simulink model "main"  (R2025b)
settings: Solver=FixedStepDiscrete  StartTime=0.0  StopTime=Inf  RelTol=1e-3  EnableMultiTasking=on
PreLoadFcn:
  | RTWConfigurationCB('preloadfcn', bdroot);
model workspace (MAT data in the model file):
  fault_count = 0
  fz_values = [0 50 100 150 200 250 300 350 400 450 500 550 ... (43 elements, 1x43)]
  k_opt_lut = [0 0 0 0 0 0 0 0 0 0 0 0 ... (4386 elements, 51x2x43)]
  mu_opt_lut = [0 0 0 0 0 0 0 0 0 0 0 0 ... (4386 elements, 51x2x43)]
undefined symbols (not defined in the file or in its folder): bit, Call, Function, ocv_lut, slope_lut, soc_lut
libraries: c2837xDlib x34, c280xlib x20, canmsglib x18, c2802xlib x12, simulink x9, slpidlib x3
(part 2 of 5)

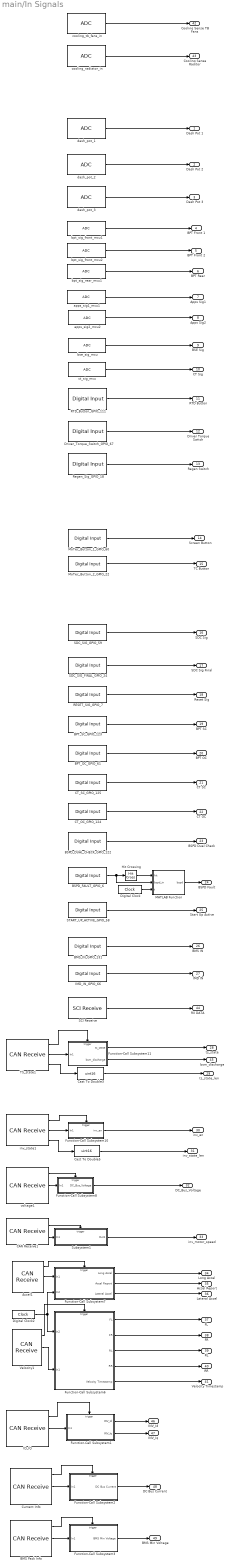
== system main/In Signals ==
  Accel1 : c280xlib/CAN Receive  chipFamily=C280x  useModule=CAN_B  mailboxNo=30  messageID=52  messageType=Standard (11-bit identifier)  enableAcceptanceFiltering=off  messageIDMask=0  sampleTime=.001  dataType=CAN_MESSAGE_TYPE  outputAction=Output last received values  initValue=0  outputMessageID=off  outputMessageLength=on  outputMessageTimeStamp=off  postInterrupt=off  interruptLine=0
  BMS Pack Info : c280xlib/CAN Receive  chipFamily=C280x  useModule=CAN_B  mailboxNo=21  messageID=237  messageType=Standard (11-bit identifier)  enableAcceptanceFiltering=off  messageIDMask=0  sampleTime=1.5  dataType=CAN_MESSAGE_TYPE  outputAction=Output last received values  initValue=2.8  outputMessageID=off  outputMessageLength=on  outputMessageTimeStamp=off  postInterrupt=off  interruptLine=0
  BMS_IN_GPIO_131 : c2837xDlib/Digital Input  GPIO_Number=GPIO128~GPIO135  GPIO_Bit0=off  GPIO_Bit1=off  GPIO_Bit2=off  GPIO_Bit3=on  GPIO_Bit4=off  GPIO_Bit5=off  GPIO_Bit6=off  GPIO_Bit7=off  sampleTime=0.01  dataType=auto  GPIO_Bit0_Qualification=Sync to SYSCLKOUT  GPIO_Bit1_Qualification=Sync to SYSCLKOUT  GPIO_Bit2_Qualification=Sync to SYSCLKOUT  GPIO_Bit3_Qualification=Sync to SYSCLKOUT  GPIO_Bit4_Qualification=Sync to SYSCLKOUT  GPIO_Bit5_Qualification=Sync to SYSCLKOUT  GPIO_Bit6_Qualification=Sync to SYSCLKOUT  GPIO_Bit7_Qualification=Sync to SYSCLKOUT  Qualification_Period=-1
  BPT_OC_GPIO_61 : c2837xDlib/Digital Input  GPIO_Number=GPIO56~GPIO63  GPIO_Bit0=off  GPIO_Bit1=off  GPIO_Bit2=off  GPIO_Bit3=off  GPIO_Bit4=off  GPIO_Bit5=on  GPIO_Bit6=off  GPIO_Bit7=off  sampleTime=0.01  dataType=auto  GPIO_Bit0_Qualification=Sync to SYSCLKOUT  GPIO_Bit1_Qualification=Sync to SYSCLKOUT  GPIO_Bit2_Qualification=Sync to SYSCLKOUT  GPIO_Bit3_Qualification=Sync to SYSCLKOUT  GPIO_Bit4_Qualification=Sync to SYSCLKOUT  GPIO_Bit5_Qualification=Sync to SYSCLKOUT  GPIO_Bit6_Qualification=Sync to SYSCLKOUT  GPIO_Bit7_Qualification=Sync to SYSCLKOUT  Qualification_Period=-1
  BPT_SC_GPIO_123 : c2837xDlib/Digital Input  GPIO_Number=GPIO120~GPIO127  GPIO_Bit0=off  GPIO_Bit1=off  GPIO_Bit2=off  GPIO_Bit3=on  GPIO_Bit4=off  GPIO_Bit5=off  GPIO_Bit6=off  GPIO_Bit7=off  sampleTime=0.01  dataType=auto  GPIO_Bit0_Qualification=Sync to SYSCLKOUT  GPIO_Bit1_Qualification=Sync to SYSCLKOUT  GPIO_Bit2_Qualification=Sync to SYSCLKOUT  GPIO_Bit3_Qualification=Sync to SYSCLKOUT  GPIO_Bit4_Qualification=Sync to SYSCLKOUT  GPIO_Bit5_Qualification=Sync to SYSCLKOUT  GPIO_Bit6_Qualification=Sync to SYSCLKOUT  GPIO_Bit7_Qualification=Sync to SYSCLKOUT  Qualification_Period=-1
  BSPD_DUAL_CHECK_GPIO_122 : c2837xDlib/Digital Input  GPIO_Number=GPIO120~GPIO127  GPIO_Bit0=off  GPIO_Bit1=off  GPIO_Bit2=on  GPIO_Bit3=off  GPIO_Bit4=off  GPIO_Bit5=off  GPIO_Bit6=off  GPIO_Bit7=off  sampleTime=0.01  dataType=auto  GPIO_Bit0_Qualification=Sync to SYSCLKOUT  GPIO_Bit1_Qualification=Sync to SYSCLKOUT  GPIO_Bit2_Qualification=Sync to SYSCLKOUT  GPIO_Bit3_Qualification=Sync to SYSCLKOUT  GPIO_Bit4_Qualification=Sync to SYSCLKOUT  GPIO_Bit5_Qualification=Sync to SYSCLKOUT  GPIO_Bit6_Qualification=Sync to SYSCLKOUT  GPIO_Bit7_Qualification=Sync to SYSCLKOUT  Qualification_Period=-1
  BSPD_FAULT_GPIO_6 : c2837xDlib/Digital Input  GPIO_Number=GPIO0~GPIO7  GPIO_Bit0=off  GPIO_Bit1=off  GPIO_Bit2=off  GPIO_Bit3=off  GPIO_Bit4=off  GPIO_Bit5=off  GPIO_Bit6=on  GPIO_Bit7=off  sampleTime=0.001  dataType=auto  GPIO_Bit0_Qualification=Sync to SYSCLKOUT  GPIO_Bit1_Qualification=Sync to SYSCLKOUT  GPIO_Bit2_Qualification=Sync to SYSCLKOUT  GPIO_Bit3_Qualification=Sync to SYSCLKOUT  GPIO_Bit4_Qualification=Sync to SYSCLKOUT  GPIO_Bit5_Qualification=Sync to SYSCLKOUT  GPIO_Bit6_Qualification=Sync to SYSCLKOUT  GPIO_Bit7_Qualification=Sync to SYSCLKOUT  Qualification_Period=-1
  CAN Receive1 : c280xlib/CAN Receive  chipFamily=C280x  useModule=CAN_B  mailboxNo=14  messageID=165  messageType=Standard (11-bit identifier)  enableAcceptanceFiltering=off  messageIDMask=0  sampleTime=0.003  dataType=CAN_MESSAGE_TYPE  outputAction=Output last received values  initValue=0  outputMessageID=off  outputMessageLength=off  outputMessageTimeStamp=off  postInterrupt=off  interruptLine=0
  CT_OC_GPIO_124 : c2837xDlib/Digital Input  GPIO_Number=GPIO120~GPIO127  GPIO_Bit0=off  GPIO_Bit1=off  GPIO_Bit2=off  GPIO_Bit3=off  GPIO_Bit4=on  GPIO_Bit5=off  GPIO_Bit6=off  GPIO_Bit7=off  sampleTime=0.01  dataType=auto  GPIO_Bit0_Qualification=Sync to SYSCLKOUT  GPIO_Bit1_Qualification=Sync to SYSCLKOUT  GPIO_Bit2_Qualification=Sync to SYSCLKOUT  GPIO_Bit3_Qualification=Sync to SYSCLKOUT  GPIO_Bit4_Qualification=Sync to SYSCLKOUT  GPIO_Bit5_Qualification=Sync to SYSCLKOUT  GPIO_Bit6_Qualification=Sync to SYSCLKOUT  GPIO_Bit7_Qualification=Sync to SYSCLKOUT  Qualification_Period=-1
  CT_SC_GPIO_125 : c2837xDlib/Digital Input  GPIO_Number=GPIO120~GPIO127  GPIO_Bit0=off  GPIO_Bit1=off  GPIO_Bit2=off  GPIO_Bit3=off  GPIO_Bit4=off  GPIO_Bit5=on  GPIO_Bit6=off  GPIO_Bit7=off  sampleTime=0.01  dataType=auto  GPIO_Bit0_Qualification=Sync to SYSCLKOUT  GPIO_Bit1_Qualification=Sync to SYSCLKOUT  GPIO_Bit2_Qualification=Sync to SYSCLKOUT  GPIO_Bit3_Qualification=Sync to SYSCLKOUT  GPIO_Bit4_Qualification=Sync to SYSCLKOUT  GPIO_Bit5_Qualification=Sync to SYSCLKOUT  GPIO_Bit6_Qualification=Sync to SYSCLKOUT  GPIO_Bit7_Qualification=Sync to SYSCLKOUT  Qualification_Period=-1
  Cast To Double3 : DataTypeConversion  OutDataTypeStr=uint16  SaturateOnIntegerOverflow=off  RndMeth=Floor
  Cast To Double5 : DataTypeConversion  OutDataTypeStr=uint16  SaturateOnIntegerOverflow=off  RndMeth=Floor
  Current Info : c280xlib/CAN Receive  chipFamily=C280x  useModule=CAN_B  mailboxNo=20  messageID=166  messageType=Standard (11-bit identifier)  enableAcceptanceFiltering=off  messageIDMask=0  sampleTime=0.003  dataType=CAN_MESSAGE_TYPE  outputAction=Reset all fields to zero  initValue=0  outputMessageID=off  outputMessageLength=on  outputMessageTimeStamp=off  postInterrupt=off  interruptLine=0
  Digital Clock : DigitalClock  SampleTime=0.001
  Digital Clock2 : DigitalClock  SampleTime=0.001
  Driver_Torque_Switch_GPIO_67 : c2837xDlib/Digital Input  GPIO_Number=GPIO64~GPIO71  GPIO_Bit0=off  GPIO_Bit1=off  GPIO_Bit2=off  GPIO_Bit3=on  GPIO_Bit4=off  GPIO_Bit5=off  GPIO_Bit6=off  GPIO_Bit7=off  sampleTime=0.1  dataType=single  GPIO_Bit0_Qualification=Sync to SYSCLKOUT  GPIO_Bit1_Qualification=Sync to SYSCLKOUT  GPIO_Bit2_Qualification=Sync to SYSCLKOUT  GPIO_Bit3_Qualification=Sync to SYSCLKOUT  GPIO_Bit4_Qualification=Sync to SYSCLKOUT  GPIO_Bit5_Qualification=Sync to SYSCLKOUT  GPIO_Bit6_Qualification=Sync to SYSCLKOUT  GPIO_Bit7_Qualification=Sync to SYSCLKOUT  Qualification_Period=-1
  Function-Call Subsystem1 : Subsystem  TreatAsAtomicUnit=on
  Function-Call Subsystem10 : Subsystem  TreatAsAtomicUnit=on
  Function-Call Subsystem11 : Subsystem  TreatAsAtomicUnit=on
  Function-Call Subsystem2 : Subsystem  TreatAsAtomicUnit=on
  Function-Call Subsystem3 : Subsystem  TreatAsAtomicUnit=on
  Function-Call Subsystem6 : Subsystem  TreatAsAtomicUnit=on
  Function-Call Subsystem7 : Subsystem  TreatAsAtomicUnit=on
  Function-Call Subsystem8 : Subsystem  TreatAsAtomicUnit=on
  Hit Crossing : HitCross  HitCrossingDirection=falling
  ID_IQ : c280xlib/CAN Receive  chipFamily=C280x  useModule=CAN_B  mailboxNo=19  messageID=168  messageType=Standard (11-bit identifier)  enableAcceptanceFiltering=off  messageIDMask=0  sampleTime=0.003  dataType=CAN_MESSAGE_TYPE  outputAction=Reset all fields to zero  initValue=0  outputMessageID=off  outputMessageLength=on  outputMessageTimeStamp=off  postInterrupt=off  interruptLine=0
  IMD_IN_GPIO_66 : c2837xDlib/Digital Input  GPIO_Number=GPIO64~GPIO71  GPIO_Bit0=off  GPIO_Bit1=off  GPIO_Bit2=on  GPIO_Bit3=off  GPIO_Bit4=off  GPIO_Bit5=off  GPIO_Bit6=off  GPIO_Bit7=off  sampleTime=0.01  dataType=auto  GPIO_Bit0_Qualification=Sync to SYSCLKOUT  GPIO_Bit1_Qualification=Sync to SYSCLKOUT  GPIO_Bit2_Qualification=Sync to SYSCLKOUT  GPIO_Bit3_Qualification=Sync to SYSCLKOUT  GPIO_Bit4_Qualification=Sync to SYSCLKOUT  GPIO_Bit5_Qualification=Sync to SYSCLKOUT  GPIO_Bit6_Qualification=Sync to SYSCLKOUT  GPIO_Bit7_Qualification=Sync to SYSCLKOUT  Qualification_Period=-1
  MATLAB Function : MATLAB Function  TreatAsAtomicUnit=on
  MoTec_Button_1_GPIO_60 : c2837xDlib/Digital Input  GPIO_Number=GPIO56~GPIO63  GPIO_Bit0=off  GPIO_Bit1=off  GPIO_Bit2=off  GPIO_Bit3=off  GPIO_Bit4=on  GPIO_Bit5=off  GPIO_Bit6=off  GPIO_Bit7=off  sampleTime=0.05  dataType=single  GPIO_Bit0_Qualification=Sync to SYSCLKOUT  GPIO_Bit1_Qualification=Sync to SYSCLKOUT  GPIO_Bit2_Qualification=Sync to SYSCLKOUT  GPIO_Bit3_Qualification=Sync to SYSCLKOUT  GPIO_Bit4_Qualification=Sync to SYSCLKOUT  GPIO_Bit5_Qualification=Sync to SYSCLKOUT  GPIO_Bit6_Qualification=Sync to SYSCLKOUT  GPIO_Bit7_Qualification=Sync to SYSCLKOUT  Qualification_Period=-1
  MoTec_Button_2_GPIO_22 : c2837xDlib/Digital Input  GPIO_Number=GPIO16~GPIO23  GPIO_Bit0=off  GPIO_Bit1=off  GPIO_Bit2=off  GPIO_Bit3=off  GPIO_Bit4=off  GPIO_Bit5=off  GPIO_Bit6=on  GPIO_Bit7=off  sampleTime=0.01  dataType=auto  GPIO_Bit0_Qualification=Sync to SYSCLKOUT  GPIO_Bit1_Qualification=Sync to SYSCLKOUT  GPIO_Bit2_Qualification=Sync to SYSCLKOUT  GPIO_Bit3_Qualification=Sync to SYSCLKOUT  GPIO_Bit4_Qualification=Sync to SYSCLKOUT  GPIO_Bit5_Qualification=Sync to SYSCLKOUT  GPIO_Bit6_Qualification=Sync to SYSCLKOUT  GPIO_Bit7_Qualification=Sync to SYSCLKOUT  Qualification_Period=-1
  RESET_SIG_GPIO_7 : c2837xDlib/Digital Input  GPIO_Number=GPIO0~GPIO7  GPIO_Bit0=off  GPIO_Bit1=off  GPIO_Bit2=off  GPIO_Bit3=off  GPIO_Bit4=off  GPIO_Bit5=off  GPIO_Bit6=off  GPIO_Bit7=on  sampleTime=0.01  dataType=auto  GPIO_Bit0_Qualification=Sync to SYSCLKOUT  GPIO_Bit1_Qualification=Sync to SYSCLKOUT  GPIO_Bit2_Qualification=Sync to SYSCLKOUT  GPIO_Bit3_Qualification=Sync to SYSCLKOUT  GPIO_Bit4_Qualification=Sync to SYSCLKOUT  GPIO_Bit5_Qualification=Sync to SYSCLKOUT  GPIO_Bit6_Qualification=Sync to SYSCLKOUT  GPIO_Bit7_Qualification=Sync to SYSCLKOUT  Qualification_Period=-1
  RTD_Button_GPIO_111 : c2837xDlib/Digital Input  GPIO_Number=GPIO104~GPIO111  GPIO_Bit0=off  GPIO_Bit1=off  GPIO_Bit2=off  GPIO_Bit3=off  GPIO_Bit4=off  GPIO_Bit5=off  GPIO_Bit6=off  GPIO_Bit7=on  sampleTime=0.1  dataType=single  GPIO_Bit0_Qualification=Sync to SYSCLKOUT  GPIO_Bit1_Qualification=Sync to SYSCLKOUT  GPIO_Bit2_Qualification=Sync to SYSCLKOUT  GPIO_Bit3_Qualification=Sync to SYSCLKOUT  GPIO_Bit4_Qualification=Sync to SYSCLKOUT  GPIO_Bit5_Qualification=Sync to SYSCLKOUT  GPIO_Bit6_Qualification=Sync to SYSCLKOUT  GPIO_Bit7_Qualification=Sync to SYSCLKOUT  Qualification_Period=-1
  Regen_Sig_GPIO_18 : c2837xDlib/Digital Input  GPIO_Number=GPIO16~GPIO23  GPIO_Bit0=off  GPIO_Bit1=off  GPIO_Bit2=on  GPIO_Bit3=off  GPIO_Bit4=off  GPIO_Bit5=off  GPIO_Bit6=off  GPIO_Bit7=off  sampleTime=0.01  dataType=single  GPIO_Bit0_Qualification=Sync to SYSCLKOUT  GPIO_Bit1_Qualification=Sync to SYSCLKOUT  GPIO_Bit2_Qualification=Sync to SYSCLKOUT  GPIO_Bit3_Qualification=Sync to SYSCLKOUT  GPIO_Bit4_Qualification=Sync to SYSCLKOUT  GPIO_Bit5_Qualification=Sync to SYSCLKOUT  GPIO_Bit6_Qualification=Sync to SYSCLKOUT  GPIO_Bit7_Qualification=Sync to SYSCLKOUT  Qualification_Period=-1
  SCI Receive : c280xlib/SCI Receive  Priority=2  sciModule=C  dataHead='S'  headerCheckMaxCount=16  dataTail='E'  dataType=int8  dataLenOptions=Length via dialog  dataDim=1  maxDataLength=1  initValue=0  errOption=Output the last received value  errValue=0  sampleTime=0.01  blockingMode=off  timeOut=inf  outputStatus=off
      settings: LibrarySourceBlock=c2802xlib/SCI Receive
  SDC_SIG_FINAL_GPIO_24 : c2837xDlib/Digital Input  GPIO_Number=GPIO24~GPIO31  GPIO_Bit0=on  GPIO_Bit1=off  GPIO_Bit2=off  GPIO_Bit3=off  GPIO_Bit4=off  GPIO_Bit5=off  GPIO_Bit6=off  GPIO_Bit7=off  sampleTime=0.001  dataType=auto  GPIO_Bit0_Qualification=Sync to SYSCLKOUT  GPIO_Bit1_Qualification=Sync to SYSCLKOUT  GPIO_Bit2_Qualification=Sync to SYSCLKOUT  GPIO_Bit3_Qualification=Sync to SYSCLKOUT  GPIO_Bit4_Qualification=Sync to SYSCLKOUT  GPIO_Bit5_Qualification=Sync to SYSCLKOUT  GPIO_Bit6_Qualification=Sync to SYSCLKOUT  GPIO_Bit7_Qualification=Sync to SYSCLKOUT  Qualification_Period=-1
  SDC_SIG_GPIO_59 : c2837xDlib/Digital Input  GPIO_Number=GPIO56~GPIO63  GPIO_Bit0=off  GPIO_Bit1=off  GPIO_Bit2=off  GPIO_Bit3=on  GPIO_Bit4=off  GPIO_Bit5=off  GPIO_Bit6=off  GPIO_Bit7=off  sampleTime=0.001  dataType=auto  GPIO_Bit0_Qualification=Sync to SYSCLKOUT  GPIO_Bit1_Qualification=Sync to SYSCLKOUT  GPIO_Bit2_Qualification=Sync to SYSCLKOUT  GPIO_Bit3_Qualification=Sync to SYSCLKOUT  GPIO_Bit4_Qualification=Sync to SYSCLKOUT  GPIO_Bit5_Qualification=Sync to SYSCLKOUT  GPIO_Bit6_Qualification=Sync to SYSCLKOUT  GPIO_Bit7_Qualification=Sync to SYSCLKOUT  Qualification_Period=-1
  START_UP_ACTIVE_GPIO_58 : c2837xDlib/Digital Input  GPIO_Number=GPIO56~GPIO63  GPIO_Bit0=off  GPIO_Bit1=off  GPIO_Bit2=on  GPIO_Bit3=off  GPIO_Bit4=off  GPIO_Bit5=off  GPIO_Bit6=off  GPIO_Bit7=off  sampleTime=0.01  dataType=auto  GPIO_Bit0_Qualification=Sync to SYSCLKOUT  GPIO_Bit1_Qualification=Sync to SYSCLKOUT  GPIO_Bit2_Qualification=Sync to SYSCLKOUT  GPIO_Bit3_Qualification=Sync to SYSCLKOUT  GPIO_Bit4_Qualification=Sync to SYSCLKOUT  GPIO_Bit5_Qualification=Sync to SYSCLKOUT  GPIO_Bit6_Qualification=Sync to SYSCLKOUT  GPIO_Bit7_Qualification=Sync to SYSCLKOUT  Qualification_Period=-1
  Subsystem1 : Subsystem
  TS_state1 : c280xlib/CAN Receive  chipFamily=C280x  useModule=CAN_B  mailboxNo=2  messageID=2  messageType=Standard (11-bit identifier)  enableAcceptanceFiltering=off  messageIDMask=0  sampleTime=.01  dataType=CAN_MESSAGE_TYPE  outputAction=Reset all fields to zero  initValue=0  outputMessageID=off  outputMessageLength=on  outputMessageTimeStamp=off  postInterrupt=off  interruptLine=0
  Velocity1 : c280xlib/CAN Receive  chipFamily=C280x  useModule=CAN_B  mailboxNo=9  messageID=51  messageType=Standard (11-bit identifier)  enableAcceptanceFiltering=off  messageIDMask=0  sampleTime=.001  dataType=CAN_MESSAGE_TYPE  outputAction=Output last received values  initValue=0  outputMessageID=off  outputMessageLength=on  outputMessageTimeStamp=off  postInterrupt=off  interruptLine=0
  apps_sig1_mcu1 : c2802xlib/ADC  blkParamProc=C2000_Type4  ADCModule=B  samplingMode=Single sample mode  ADCResolution=12-bit (Single-ended input)  ADC29xResolution=12-bit  ADCMode=Single-ended input  useSOC1=SOC6  useSOC2=SOC0_SOC1  SOCAcquisitionWindow=60  SOCTriggerSource=Software  SOCInterruptTrigger=No ADCINT  Ts=0.001  dType=uint16  postInterrupt=off  interruptSel=ADCINT1  ADCINTContinuous=on  endma=off  chdma=1  conv1=ADCINA0  conv2=ADCINA0 and ADCINB0  conv1_Type4=ADCIN3  conv2_Type4=ADCIN0 and ADCIN1
  apps_sig2_mcu2 : c2802xlib/ADC  blkParamProc=C2000_Type4  ADCModule=C  samplingMode=Single sample mode  ADCResolution=12-bit (Single-ended input)  ADC29xResolution=12-bit  ADCMode=Single-ended input  useSOC1=SOC7  useSOC2=SOC0_SOC1  SOCAcquisitionWindow=60  SOCTriggerSource=Software  SOCInterruptTrigger=No ADCINT  Ts=0.001  dType=uint16  postInterrupt=off  interruptSel=ADCINT1  ADCINTContinuous=on  endma=off  chdma=1  conv1=ADCINA0  conv2=ADCINA0 and ADCINB0  conv1_Type4=ADCIN3  conv2_Type4=ADCIN0 and ADCIN1
  bpt_sig_front_mcu1 : c2802xlib/ADC  blkParamProc=C2000_Type4  ADCModule=B  samplingMode=Single sample mode  ADCResolution=12-bit (Single-ended input)  ADC29xResolution=12-bit  ADCMode=Single-ended input  useSOC1=SOC3  useSOC2=SOC0_SOC1  SOCAcquisitionWindow=60  SOCTriggerSource=Software  SOCInterruptTrigger=No ADCINT  Ts=0.001  dType=uint16  postInterrupt=off  interruptSel=ADCINT1  ADCINTContinuous=on  endma=off  chdma=1  conv1=ADCINA0  conv2=ADCINA0 and ADCINB0  conv1_Type4=ADCIN4  conv2_Type4=ADCIN0 and ADCIN1
  bpt_sig_front_mcu2 : c2802xlib/ADC  blkParamProc=C2000_Type4  ADCModule=B  samplingMode=Single sample mode  ADCResolution=12-bit (Single-ended input)  ADC29xResolution=12-bit  ADCMode=Single-ended input  useSOC1=SOC4  useSOC2=SOC0_SOC1  SOCAcquisitionWindow=60  SOCTriggerSource=Software  SOCInterruptTrigger=No ADCINT  Ts=0.001  dType=uint16  postInterrupt=off  interruptSel=ADCINT1  ADCINTContinuous=on  endma=off  chdma=1  conv1=ADCINA0  conv2=ADCINA0 and ADCINB0  conv1_Type4=ADCIN2  conv2_Type4=ADCIN0 and ADCIN1
  bpt_sig_rear_mcu1 : c2802xlib/ADC  blkParamProc=C2000_Type4  ADCModule=C  samplingMode=Single sample mode  ADCResolution=12-bit (Single-ended input)  ADC29xResolution=12-bit  ADCMode=Single-ended input  useSOC1=SOC5  useSOC2=SOC0_SOC1  SOCAcquisitionWindow=60  SOCTriggerSource=Software  SOCInterruptTrigger=No ADCINT  Ts=0.001  dType=uint16  postInterrupt=off  interruptSel=ADCINT1  ADCINTContinuous=on  endma=off  chdma=1  conv1=ADCINA0  conv2=ADCINA0 and ADCINB0  conv1_Type4=ADCIN2  conv2_Type4=ADCIN0 and ADCIN1
  bse_sig_mcu : c2802xlib/ADC  blkParamProc=C2000_Type4  ADCModule=A  samplingMode=Single sample mode  ADCResolution=12-bit (Single-ended input)  ADC29xResolution=12-bit  ADCMode=Single-ended input  useSOC1=SOC8  useSOC2=SOC0_SOC1  SOCAcquisitionWindow=60  SOCTriggerSource=Software  SOCInterruptTrigger=No ADCINT  Ts=0.01  dType=uint16  postInterrupt=off  interruptSel=ADCINT1  ADCINTContinuous=on  endma=off  chdma=1  conv1=ADCINA0  conv2=ADCINA0 and ADCINB0  conv1_Type4=ADCIN3  conv2_Type4=ADCIN0 and ADCIN1
  cooling_radiator_in : c2802xlib/ADC  blkParamProc=C2000_Type4  ADCModule=A  samplingMode=Single sample mode  ADCResolution=12-bit (Single-ended input)  ADC29xResolution=12-bit  ADCMode=Single-ended input  useSOC1=SOC11  useSOC2=SOC0_SOC1  SOCAcquisitionWindow=60  SOCTriggerSource=Software  SOCInterruptTrigger=ADCINT1  Ts=1  dType=uint16  postInterrupt=off  interruptSel=ADCINT1  ADCINTContinuous=on  endma=off  chdma=1  conv1=ADCINA0  conv2=ADCINA0 and ADCINB0  conv1_Type4=ADCIN5  conv2_Type4=ADCIN0 and ADCIN1
  cooling_tb_fans_in : c2802xlib/ADC  blkParamProc=C2000_Type4  ADCModule=B  samplingMode=Single sample mode  ADCResolution=12-bit (Single-ended input)  ADC29xResolution=12-bit  ADCMode=Single-ended input  useSOC1=SOC10  useSOC2=SOC0_SOC1  SOCAcquisitionWindow=60  SOCTriggerSource=Software  SOCInterruptTrigger=No ADCINT  Ts=1  dType=uint16  postInterrupt=off  interruptSel=ADCINT1  ADCINTContinuous=on  endma=off  chdma=1  conv1=ADCINA0  conv2=ADCINA0 and ADCINB0  conv1_Type4=ADCIN5  conv2_Type4=ADCIN0 and ADCIN1
  ct_sig_mcu : c2802xlib/ADC  blkParamProc=C2000_Type4  ADCModule=A  samplingMode=Single sample mode  ADCResolution=12-bit (Single-ended input)  ADC29xResolution=12-bit  ADCMode=Single-ended input  useSOC1=SOC9  useSOC2=SOC0_SOC1  SOCAcquisitionWindow=60  SOCTriggerSource=Software  SOCInterruptTrigger=No ADCINT  Ts=0.01  dType=uint16  postInterrupt=off  interruptSel=ADCINT1  ADCINTContinuous=on  endma=off  chdma=1  conv1=ADCINA0  conv2=ADCINA0 and ADCINB0  conv1_Type4=ADCIN2  conv2_Type4=ADCIN0 and ADCIN1
  dash_pot_1 : c2802xlib/ADC  blkParamProc=C2000_Type4  ADCModule=A  samplingMode=Single sample mode  ADCResolution=12-bit (Single-ended input)  ADC29xResolution=12-bit  ADCMode=Single-ended input  useSOC1=SOC0  useSOC2=SOC0_SOC1  SOCAcquisitionWindow=60  SOCTriggerSource=Software  SOCInterruptTrigger=No ADCINT  Ts=0.05  dType=uint16  postInterrupt=off  interruptSel=ADCINT1  ADCINTContinuous=on  endma=off  chdma=1  conv1=ADCINA0  conv2=ADCINA0 and ADCINB0  conv1_Type4=ADCIN14  conv2_Type4=ADCIN0 and ADCIN1
  dash_pot_2 : c2802xlib/ADC  blkParamProc=C2000_Type4  ADCModule=A  samplingMode=Single sample mode  ADCResolution=12-bit (Single-ended input)  ADC29xResolution=12-bit  ADCMode=Single-ended input  useSOC1=SOC1  useSOC2=SOC0_SOC1  SOCAcquisitionWindow=60  SOCTriggerSource=Software  SOCInterruptTrigger=No ADCINT  Ts=0.05  dType=uint16  postInterrupt=off  interruptSel=ADCINT1  ADCINTContinuous=on  endma=off  chdma=1  conv1=ADCINA0  conv2=ADCINA0 and ADCINB0  conv1_Type4=ADCIN4  conv2_Type4=ADCIN0 and ADCIN1
  dash_pot_3 : c2802xlib/ADC  blkParamProc=C2000_Type4  ADCModule=A  samplingMode=Single sample mode  ADCResolution=12-bit (Single-ended input)  ADC29xResolution=12-bit  ADCMode=Single-ended input  useSOC1=SOC2  useSOC2=SOC0_SOC1  SOCAcquisitionWindow=60  SOCTriggerSource=Software  SOCInterruptTrigger=No ADCINT  Ts=0.05  dType=uint16  postInterrupt=off  interruptSel=ADCINT1  ADCINTContinuous=on  endma=off  chdma=1  conv1=ADCINA0  conv2=ADCINA0 and ADCINB0  conv1_Type4=ADCIN1  conv2_Type4=ADCIN0 and ADCIN1
  inv_state1 : c280xlib/CAN Receive  chipFamily=C280x  useModule=CAN_B  mailboxNo=5  messageID=170  messageType=Standard (11-bit identifier)  enableAcceptanceFiltering=off  messageIDMask=0  sampleTime=.01  dataType=CAN_MESSAGE_TYPE  outputAction=Reset all fields to zero  initValue=0  outputMessageID=off  outputMessageLength=on  outputMessageTimeStamp=off  postInterrupt=off  interruptLine=0
  voltage1 : c280xlib/CAN Receive  chipFamily=C280x  useModule=CAN_B  mailboxNo=15  messageID=167  messageType=Standard (11-bit identifier)  enableAcceptanceFiltering=off  messageIDMask=0  sampleTime=0.003  dataType=CAN_MESSAGE_TYPE  outputAction=Reset all fields to zero  initValue=0  outputMessageID=off  outputMessageLength=on  outputMessageTimeStamp=off  postInterrupt=off  interruptLine=0
  Dash Pot 1 : Outport
  Dash Pot 2 : Outport  Port=2
  Dash Pot 3 : Outport  Port=3
  BPT Front 1 : Outport  Port=4
  BPT Front 2 : Outport  Port=5
  BPT Rear : Outport  Port=6
  Apps Sig1 : Outport  Port=7
  Apps Sig2 : Outport  Port=8
  BSE Sig : Outport  Port=9
  CT Sig : Outport  Port=10
  RTD Button : Outport  Port=11
  Driver Torque Switch : Outport  Port=12
  Regen Switch : Outport  Port=13
  Screen Button : Outport  Port=14
  TC Button : Outport  Port=15
  SDC Sig : Outport  Port=16
  SDC Sig Final : Outport  Port=17
  Reset Sig : Outport  Port=18
  BPT SC : Outport  Port=19
  BPT OC : Outport  Port=20
  CT SC : Outport  Port=21
  CT OC : Outport  Port=22
  BSPD Dual Check : Outport  Port=23
  BSPD Fault : Outport  Port=24
  Start Up Active : Outport  Port=25
  BMS IN : Outport  Port=26
  IMD IN : Outport  Port=27
  ts_state : Outport  Port=28
  ts_state_len : Outport  Port=29
  inv_en : Outport  Port=30
  inv_state_len : Outport  Port=31
  DC_Bus_Voltage : Outport  Port=32
  inv_motor_speed : Outport  Port=33
  Long Accel : Outport  Port=34
  Accel Report : Outport  Port=35
  Lateral Accel : Outport  Port=36
  FL : Outport  Port=37
  FR : Outport  Port=38
  RL : Outport  Port=39
  RR : Outport  Port=40
  Velocity Timestamp : Outport  Port=41
  Cooling Sense TB Fans : Outport  Port=42
  Cooling Sense Raditor : Outport  Port=43
  RX DATA : Outport  Port=44
  bsm_discharge : Outport  Port=45
  INV_Id : Outport  Port=46
  INV_Iq : Outport  Port=47
  DC Bus Current : Outport  Port=48
  BMS Min Voltage : Outport  Port=49
  wires:
  apps_sig2_mcu2/1 -> Apps Sig2/1
  voltage1/2 -> Function-Call Subsystem8/1(In1)
  voltage1/1 -> Function-Call Subsystem8/Trigger
  CT_OC_GPIO_124/1 -> CT OC/1
  CAN Receive1/2 -> Subsystem1/1(In1)
  Function-Call Subsystem7/2(Accel Report) -> Accel Report/1
  Digital Clock2/1 -> Function-Call Subsystem6/1(In2), Function-Call Subsystem7/2(In2)
  dash_pot_1/1 -> Dash Pot 1/1
  TS_state1/2 -> Function-Call Subsystem11/1(In1)
  Function-Call Subsystem11/1(ts_state) -> ts_state/1
  inv_state1/1 -> Function-Call Subsystem10/Trigger
  inv_state1/3 -> Cast To Double5/1
  RTD_Button_GPIO_111/1 -> RTD Button/1
  Velocity1/1 -> Function-Call Subsystem6/Trigger
  Cast To Double3/1 -> ts_state_len/1
  BSPD_DUAL_CHECK_GPIO_122/1 -> BSPD Dual Check/1
  Accel1/2 -> Function-Call Subsystem7/1(In1)
  TS_state1/1 -> Function-Call Subsystem11/Trigger
  START_UP_ACTIVE_GPIO_58/1 -> Start Up Active/1
  Accel1/1 -> Function-Call Subsystem7/Trigger
  MoTec_Button_2_GPIO_22/1 -> TC Button/1
  Velocity1/2 -> Function-Call Subsystem6/2(In1)
  Function-Call Subsystem7/3(Lateral Accel) -> Lateral Accel/1
  Function-Call Subsystem7/1(Long Accel) -> Long Accel/1
  TS_state1/3 -> Cast To Double3/1
  inv_state1/2 -> Function-Call Subsystem10/1(In1)
  SDC_SIG_FINAL_GPIO_24/1 -> SDC Sig Final/1
  CAN Receive1/1 -> Subsystem1/Trigger
  Function-Call Subsystem6/5(Velocity Timestamp) -> Velocity Timestamp/1
  bse_sig_mcu/1 -> BSE Sig/1
  MoTec_Button_1_GPIO_60/1 -> Screen Button/1
  IMD_IN_GPIO_66/1 -> IMD IN/1
  dash_pot_2/1 -> Dash Pot 2/1
  BPT_OC_GPIO_61/1 -> BPT OC/1
  CT_SC_GPIO_125/1 -> CT SC/1
  bpt_sig_front_mcu2/1 -> BPT Front 2/1
  ct_sig_mcu/1 -> CT Sig/1
  Function-Call Subsystem6/1(FL) -> FL/1
  Function-Call Subsystem6/4(RR) -> RR/1
  Function-Call Subsystem6/2(FR) -> FR/1
  BPT_SC_GPIO_123/1 -> BPT SC/1
  dash_pot_3/1 -> Dash Pot 3/1
  BSPD_FAULT_GPIO_6/1 -> MATLAB Function/2(bspd_in), Hit Crossing/1
  BMS_IN_GPIO_131/1 -> BMS IN/1
  Function-Call Subsystem10/1(inv_en) -> inv_en/1
  Driver_Torque_Switch_GPIO_67/1 -> Driver Torque Switch/1
  apps_sig1_mcu1/1 -> Apps Sig1/1
  bpt_sig_front_mcu1/1 -> BPT Front 1/1
  Function-Call Subsystem8/1(DC_Bus_Voltage) -> DC_Bus_Voltage/1
  Subsystem1/1(Out1) -> inv_motor_speed/1
  SDC_SIG_GPIO_59/1 -> SDC Sig/1
  bpt_sig_rear_mcu1/1 -> BPT Rear/1
  Cast To Double5/1 -> inv_state_len/1
  Function-Call Subsystem6/3(RL) -> RL/1
  RESET_SIG_GPIO_7/1 -> Reset Sig/1
  Regen_Sig_GPIO_18/1 -> Regen Switch/1
  cooling_tb_fans_in/1 -> Cooling Sense TB Fans/1
  cooling_radiator_in/1 -> Cooling Sense Raditor/1
  SCI Receive/1 -> RX DATA/1
  Function-Call Subsystem11/2(bsm_discharge) -> bsm_discharge/1
  ID_IQ/1 -> Function-Call Subsystem1/Trigger
  ID_IQ/2 -> Function-Call Subsystem1/1(In1)
  Function-Call Subsystem1/1(INV_Id) -> INV_Id/1
  Function-Call Subsystem1/2(INV_Iq) -> INV_Iq/1
  Hit Crossing/1 -> MATLAB Function/1(hit)
  Digital Clock/1 -> MATLAB Function/3(t)
  MATLAB Function/1(bspd) -> BSPD Fault/1
  Current Info/2 -> Function-Call Subsystem2/1(In1)
  Current Info/1 -> Function-Call Subsystem2/Trigger
  Function-Call Subsystem2/1(DC Bus Current) -> DC Bus Current/1
  Function-Call Subsystem3/1(BMS Min Voltage) -> BMS Min Voltage/1
  BMS Pack Info/1 -> Function-Call Subsystem3/Trigger
  BMS Pack Info/2 -> Function-Call Subsystem3/1(In1)

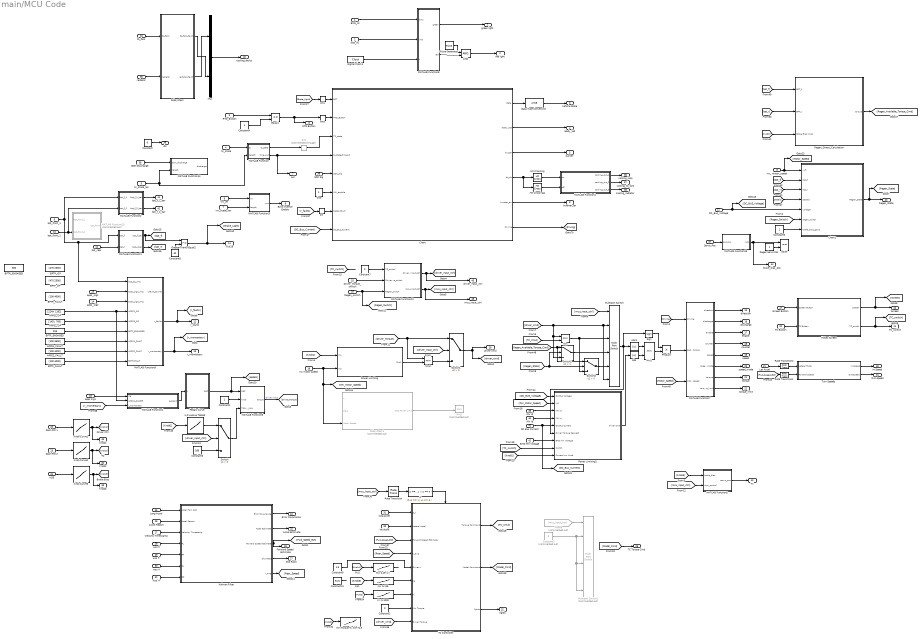
== system main/MCU Code ==
  BMS_IN : Inport
  IMD_IN : Inport  Port=2
  RTD_Button : Inport  Port=3
  ts_state : Inport  Port=4
  ts_state_len : Inport  Port=5
  inv_en : Inport  Port=6
  inv_state_len : Inport  Port=7
  inv_ motor_speed : Inport  Port=8
  bpt_front_1 : Inport  Port=9
  bpt_front_2 : Inport  Port=10
  bpt_rear : Inport  Port=11
  DC_Bus_Voltage : Inport  Port=12
  apps_sig1 : Inport  Port=13
  apps_sig2 : Inport  Port=14
  Driver_Torque_switch : Inport  Port=15
  Regen_switch : Inport  Port=16
  Screen Button : Inport  Port=17
  inv motor speed : Inport  Port=18
  apps sig1 : Inport  Port=19
  TC Button : Inport  Port=20
  Lat Accel : Inport  Port=21
  Dash Pot 1 : Inport  Port=22
  Dash Pot 2 : Inport  Port=23
  In26 : Inport  Port=24
  Long Accel : Inport  Port=25
  Accel Report : Inport  Port=26
  Velocity Timestamp : Inport  Port=27
  wss fl : Inport  Port=28
  wss fr : Inport  Port=29
  wss rl : Inport  Port=30
  long accel : Inport  Port=31
  wss rr : Inport  Port=32
  lat accel : Inport  Port=33
  tb_fans : Inport  Port=34
  radiator : Inport  Port=35
  SDC Sig : Inport  Port=36
  Servo_Pos : Inport  Port=37
  BSM Discharge : Inport  Port=38
  INV Id : Inport  Port=39
  INV Iq : Inport  Port=40
  DC Bus Current : Inport  Port=41
  BMS Min Voltage : Inport  Port=42
  1-D Lookup Table3 : Lookup_n-D  NumberOfTableDimensions=1  BreakpointsForDimension1=[1;10]  Table=[20;166]  ExtrapMethod=Clip  InternalRulePriority=Speed  RndMeth=Simplest
  AND : Logic  IconShape=distinctive  AllPortsSameDT=off  OutDataTypeStr=boolean
  APPS1_FAULT : Constant  Value=[100 3500]  VectorParams1D=off
  APPS1_OP : Constant  Value="[2249  1262]"  VectorParams1D=off
  APPS2_FAULT : Constant  Value=[100 4000]  VectorParams1D=off
  APPS2_OP : Constant  Value="[1431  760]"  VectorParams1D=off
  Abs : Abs  SaturateOnIntegerOverflow=off
  Abs1 : Abs  SaturateOnIntegerOverflow=off
  BPTF_ENGAGED : Constant  Value=913  VectorParams1D=off
  BPTF_FAULT : Constant  Value=[100 4000]  VectorParams1D=off
  BPTF_OP : Constant  Value=[475 2300]  VectorParams1D=off
  BPTR_ENGAGED : Constant  Value=600  VectorParams1D=off
  BPTR_FAULT : Constant  Value=[100 4000]  VectorParams1D=off
  BPTR_OP : Constant  Value=[475 2300]  VectorParams1D=off
  Chart : Stateflow chart  TreatAsAtomicUnit=on  SystemSampleTime=0.01
      settings: RTWSystemCode=Inline  RTWFcnNameOpts=Use subsystem name  RTWFileNameOpts=Use subsystem name  PortSchema="{\"entries\":[{\"content\":{\"sides\":[{\"content\":{\"connectorIds\":[\"In1\",\"In2\",\"In7\",\"In4\",\"In5\",\"In6\",\"In3\",\"In8\"]},\"type\":\"ConnectorPlacement.EquallySpacedRectSide\",\"uuid\":\"e489c846-491e-4e82-9c5f-b669d7c96954\"},{\"content\":{\"connectorIds\":[\"Out1\",\"Out2\",\"Out3\",\"Out4\",\"Out5\",\"Out6\"],\"side\":\"RIGHT\"},\"type\":\"ConnectorPlacement.EquallySpacedRectSide\",\"uuid\":\"cbb46da5-6eb6-44f9-baf3-a24ec6c96225\"},{\"content\":{\"side\":\"TOP\"},\"type\":\"ConnectorPlacement.EquallySpacedRectSide\",\"uuid\":\"c6202e3b-aafb-4b81-a309-4cc98c9bb853\"},{\"content\":{\"side\":\"BOTTOM\"},\"type\":\"ConnectorPlacement.EquallySpacedRectSide\",\"uuid\":\"d6a20d7c-ea9b-4afd-8884-952a45f498ea\"}]},\"type\":\"ConnectorPlacement.EquallySpacedConnector\",\"uuid\":\"7c3bea70-19b9-40c4-b7cb-79b1c3f0d3c0\"}],\"packageUris\":[\"http://schema.mathworks.com/mf0/Connector/R2020b\"],\"version\":\"1.0\"}"
  Chart1 : Stateflow chart  TreatAsAtomicUnit=on
  Constant : Constant  Value=0
  Constant1 : Constant
  Constant10 : Constant  Value=51.5
  Constant2 : Constant  Value=0
  Constant3 : Constant  Commented=on  Value=0
  Constant4 : Constant  OutDataTypeStr=single
  Constant5 : Constant  Value=166
  Constant6 : Constant  OutDataTypeStr=boolean
  Constant7 : Constant  Value=0
  Constant8 : Constant  Value=40
  Constant9 : Constant  Value=1.5
  Data Type Conversion : DataTypeConversion  OutDataTypeStr=uint8  SaturateOnIntegerOverflow=off  RndMeth=Floor
  Digital Clock1 : DigitalClock  SampleTime=0.01
  Equal : RelationalOperator  Operator===  OutDataTypeStr=boolean  RndMeth=Simplest  InputSameDT=off
  Equal1 : RelationalOperator  Operator===  OutDataTypeStr=Inherit: Inherit via back propagation  RndMeth=Simplest  InputSameDT=off
  From9 : From  Commented=on  GotoTag=mcu_input_ctrl
  GreaterThanOrEqual2 : RelationalOperator  OutDataTypeStr=boolean  RndMeth=Simplest  InputSameDT=off
  Hit Crossing : HitCross  HitCrossingOffset=1  HitCrossingDirection=rising
  Hit Crossing1 : HitCross  HitCrossingOffset=1  HitCrossingDirection=falling
  If : If  IfExpression=u1 == 1 | u1 == 3  ShowElse=off
  Kalman Filter : Subsystem
  Ki: 0-1000 : Lookup_n-D  NumberOfTableDimensions=1  BreakpointsForDimension1=[1 10]  Table=[0 900]  ExtrapMethod=Clip  InternalRulePriority=Speed  RndMeth=Simplest
  Knob Curve1 : Lookup_n-D  NumberOfTableDimensions=1  BreakpointsForDimension1=[0;280;640;1200;1480;1940;2440;2960;3500;4080]  BreakpointsForDimension1DataTypeStr=uint16  BeginIndexSearchUsingPreviousIndexResult=on  Table=[1;2;3;4;5;6;7;8;9;10]  TableDataTypeStr=double  InterpMethod=Nearest  ExtrapMethod=Clip  DiagnosticForOutOfRangeInput=Warning  UseLastTableValue=on  InternalRulePriority=Speed  OutDataTypeStr=double  RndMeth=Simplest
  Knob Curve2 : Lookup_n-D  NumberOfTableDimensions=1  BreakpointsForDimension1=[0;180;640;1040;1480;1920;2420;2920;3480;4080]  BreakpointsForDimension1DataTypeStr=uint16  BeginIndexSearchUsingPreviousIndexResult=on  Table=[1;2;3;4;5;6;7;8;9;10]  TableDataTypeStr=double  InterpMethod=Nearest  ExtrapMethod=Clip  DiagnosticForOutOfRangeInput=Warning  UseLastTableValue=on  InternalRulePriority=Speed  OutDataTypeStr=double  RndMeth=Simplest
  Knob Curve3 : Lookup_n-D  NumberOfTableDimensions=1  BreakpointsForDimension1=[0;140;600;980;1380;1780;2220;2660;3240;3920]  BreakpointsForDimension1DataTypeStr=uint16  BeginIndexSearchUsingPreviousIndexResult=on  Table=[1;2;3;4;5;6;7;8;9;10]  TableDataTypeStr=double  InterpMethod=Nearest  ExtrapMethod=Clip  DiagnosticForOutOfRangeInput=Warning  UseLastTableValue=on  InternalRulePriority=Speed  OutDataTypeStr=double  RndMeth=Simplest
  Kp: 0-115 : Lookup_n-D  NumberOfTableDimensions=1  BreakpointsForDimension1=[1 10]  Table=[0 115]  InternalRulePriority=Speed  RndMeth=Simplest
  MATLAB Function : MATLAB Function  TreatAsAtomicUnit=on
  MATLAB Function1 : MATLAB Function  TreatAsAtomicUnit=on
  MATLAB Function10 : MATLAB Function  Commented=on  TreatAsAtomicUnit=on
  MATLAB Function11 : MATLAB Function  TreatAsAtomicUnit=on
  MATLAB Function12 : MATLAB Function  TreatAsAtomicUnit=on
  MATLAB Function13 : MATLAB Function  TreatAsAtomicUnit=on
  MATLAB Function14 : MATLAB Function  TreatAsAtomicUnit=on
  MATLAB Function2 : MATLAB Function  TreatAsAtomicUnit=on
  MATLAB Function3 : MATLAB Function  TreatAsAtomicUnit=on
  MATLAB Function4 : MATLAB Function  TreatAsAtomicUnit=on
  MATLAB Function5 : MATLAB Function  TreatAsAtomicUnit=on
  MATLAB Function6 : MATLAB Function  TreatAsAtomicUnit=on
  MATLAB Function7 : MATLAB Function  TreatAsAtomicUnit=on
  MATLAB Function8 : MATLAB Function  TreatAsAtomicUnit=on
  MATLAB Function9 : MATLAB Function  TreatAsAtomicUnit=on
  Min : MinMax  Inputs=2
  Min Torque %: 0.0-72.5 : Lookup_n-D  NumberOfTableDimensions=1  BreakpointsForDimension1=[1 10]  Table=[0 0.725]  InternalRulePriority=Speed  RndMeth=Simplest
  Min1 : MinMax  Inputs=2
  Min2 : MinMax  Inputs=2
  Min3 : MinMax  Commented=on  Inputs=2
  Motec Screen : Subsystem
  Mu: 0.45-1.7 : Lookup_n-D  NumberOfTableDimensions=1  BreakpointsForDimension1=[1 10]  Table=[0.45 1.7]  ExtrapMethod=Clip  InternalRulePriority=Speed  RndMeth=Simplest
  Multiport Switch : MultiPortSwitch  DataPortOrder=Zero-based contiguous  Inputs=4  DataPortForDefault=Additional data port  zeroidx=on  SaturateOnIntegerOverflow=off  InputSameDT=off
  Multiport Switch2 : MultiPortSwitch  Commented=on  DataPortOrder=Zero-based contiguous  Inputs=4  DataPortForDefault=Additional data port  zeroidx=on  SaturateOnIntegerOverflow=off  InputSameDT=off
  Mux : Mux  Inputs=2
  One : Constant  OutDataTypeStr=Inherit: Inherit via back propagation
  Pedals Curve : Subsystem
  Power Limiting : Subsystem
  Power Limiting1 : Subsystem
  Product : Product
  Pulse Generator : DiscretePulseGenerator  PulseType=Time based  Period=1/4  PulseWidth=50
  RT : RateTransition  OutPortSampleTime=0.01
  RT2 : RateTransition  Commented=through  OutPortSampleTime=0.01
  RT3 : RateTransition  OutPortSampleTime=0.01
  RT4 : RateTransition  OutPortSampleTime=0.01
  Rate Transition : RateTransition  OutPortSampleTime=0.001
  Rate Transition1 : RateTransition  OutPortSampleTime=0.01
  Rate Transition2 : RateTransition  OutPortSampleTime=0.01
  Regen Servo Pos : Constant
  Regen_Direct_Calculation : Subsystem
  Sign : Signum
  Subsystem : Subsystem
  Subsystem1 : Subsystem  Commented=on
  Switch : Switch  Criteria=u2 > Threshold  SaturateOnIntegerOverflow=off  InputSameDT=off
  Switch1 : Switch  Criteria=u2 > Threshold  SaturateOnIntegerOverflow=off  InputSameDT=off
  Switch2 : Switch  Criteria=u2 > Threshold  Threshold=1  SaturateOnIntegerOverflow=off  InputSameDT=off
  Switch3 : Switch  Criteria=u2 > Threshold  SaturateOnIntegerOverflow=off  InputSameDT=off
  TC Controller : Subsystem
  Turn Speeds : Subsystem
  green light : Outport
  red light : Outport  Port=2
  Vehicle State : Outport  Port=3
  ready_led : Outport  Port=4
  buzzer : Outport  Port=5
  RTD Button : Outport  Port=6
  out : Outport  Port=7
  inverter_en : Outport  Port=8
  Echo Inverter Enable : Outport  Port=9
  Screen : Outport  Port=10
  TC_switch : Outport  Port=11
  r_faults : Outport  Port=12
  r_momentary : Outport  Port=13
  Out18 : Outport  Port=14
  direction : Outport  Port=15
  discharge : Outport  Port=16
  enable : Outport  Port=17
  counter : Outport  Port=18
  speed : Outport  Port=19
  speed_mode : Outport  Port=20
  torque : Outport  Port=21
  torque_limit : Outport  Port=22
  Regen_State : Outport  Port=23
  Error Covariance : Outport  Port=24
  Accel Estimate : Outport  Port=25
  Forward Speed Estimate : Outport  Port=26
  Slip Ratio : Outport  Port=27
  driver cmd : Outport  Port=28
  TC Torque Cmd : Outport  Port=29
  In-Speed : Outport  Port=30
  Out-Speed : Outport  Port=31
  lights : Outport  Port=32
  Knob1 : Outport  Port=33
  Knob2 : Outport  Port=34
  Knob3 : Outport  Port=35
  cooling_loop : Outport  Port=36
  cooling_tb_fans : Outport  Port=37
  cooling_radiator : Outport  Port=38
  dis : Outport  Port=39
  cooling_faults : Outport  Port=40
  bpt_f_1_bar : Outport  Port=41
  bpt_f_2_bar : Outport  Port=42
  TX : Outport  Port=43
  brake_bias_pos : Outport  Port=44
  driver_input_ctrl : Outport  Port=45
  mcu_input_ctrl : Outport  Port=46
  wires:
  BPTF_ENGAGED/1 -> MATLAB Function9/6(BPTF_ENGAGED)
  [r_faults] -> RT/1
  Constant10/1 -> ?
  Motec Screen/1(Screen) -> [Screen], Screen/1
  [driver_cmd] -> Min/1, Switch2/3, Multiport Switch/6, Multiport Switch/2
  [Driver_Torque] -> Min2/1, Switch1/1
  Constant9/1 -> TC Controller/5(Driver u)
  RT/1 -> Chart/3(Pedal_Fault)
  [Motor_Speed] -> MATLAB Function7/3(motor_speed)
  [driving] -> MATLAB Function7/1(driving)
  TC Button/1 -> Motec Screen/2(TC Button)
  APPS1_OP/1 -> MATLAB Function9/4(APPS1_OP), MATLAB Function4/2(APPS1_RANGE)
  BPTF_FAULT/1 -> MATLAB Function9/9(BPTF_FAULT)
  apps_sig2/1 -> MATLAB Function9/3(apps_sig2_mcu)
  [Rear_Speed] -> TC Controller/4(v_avg)
  [Regen_State] -> Switch3/2, Switch2/2
  APPS1_FAULT/1 -> MATLAB Function9/7(APPS1_FAULT)
  Power Limiting/1(Out1) -> Min2/2
  Constant3/1 -> Multiport Switch2/4, Multiport Switch2/6, Multiport Switch2/2
  [Fwd_Speed_Est] -> TC Controller/3(Forward Speed Estimate)
  One/1 -> Chart/6(INV_enable)
  RT2/1 -> Chart/7(TS_state)
  [mcu_input_ctrl] -> Rate Transition/1
  MATLAB Function11/1(bpt_f_bar) -> GreaterThanOrEqual2/1, [bpt_f]
  Kalman Filter/2(Accel Estimate) -> Accel Estimate/1
  1-D Lookup Table3/1 -> Switch/1
  Equal1/1 -> RTD Button/1, RT3/1
  Knob Curve3/1 -> Knob3/1, [Knob3]
  [bpt_f] -> Regen_Direct_Calculation/1(BPT_f)
  [Knob2] -> Ki: 0-1000/1
  Digital Clock1/1 -> MATLAB Function8/3(t)
  Constant1/1 -> MATLAB Function6/2(knob)
  MATLAB Function4/1(percent) -> Pedals Curve/1(u)
  TC Controller/2(Model Command) -> [Model_Cmd]
  bpt_rear/1 -> MATLAB Function11/2(bpt_r)
  inv_ motor_speed/1 -> [Motor_Speed], Chart1/1(v_fr)
  [driver_input_ctrl] -> Switch1/2
  Switch2/1 -> Multiport Switch/4
  long accel/1 -> TC Controller/1(a_x)
  MATLAB Function9/3(r_momentary) -> [r_momentary], r_momentary/1
  [Regen_Switch] -> Chart1/6(regen_switch)
  RT4/1 -> Chart/1(BPT)
  [TC_switch] -> ?
  Knob Curve2/1 -> Knob2/1, [Knob2]
  From9/1 -> Multiport Switch2/1
  APPS2_FAULT/1 -> MATLAB Function9/8(APPS2_FAULT)
  Constant8/1 -> GreaterThanOrEqual2/2
  Kalman Filter/5(v_avg) -> [Rear_Speed]
  apps sig1/1 -> MATLAB Function4/1(sig)
  wss rr/1 -> Kalman Filter/7(RR)
  [Regen_Available_Torque_Cmd] -> Switch3/1, Switch2/1
  Multiport Switch/1 -> Power Limiting1/6(Driver Torque Request), Sign/1, Abs1/1
  bpt_front_2/1 -> MATLAB Function10/2(bpt_front_2), MATLAB Function2/2(bpt_f_2)
  [mcu_input_ctrl] -> Multiport Switch/1
  Pulse Generator/1 -> AND/1
  Data Type Conversion/1 -> Vehicle State/1
  [r_momentary] -> MATLAB Function4/3(r_momentary)
  Pedals Curve/1(ped) -> [pedals], MATLAB Function6/1(ped)
  Knob Curve1/1 -> Knob1/1, [Knob1]
  MATLAB Function12/1(driver_input_ctrl) -> driver_input_ctrl/1, [driver_input_ctrl]
  [driver_cmd] -> TC Controller/9(Driver Torque)
  [Knob3] -> Kp: 0-115/1
  MATLAB Function3/1(out) -> Echo Inverter Enable/1
  Min/1 -> Switch3/3, Multiport Switch/3
  Motec Screen/2(TC_switch) -> [TC_switch], TC_switch/1
  wss fr/1 -> Kalman Filter/5(FR)
  TC Controller/1(Torque Command) -> [TC_Cmd]
  Chart/1(state) -> Data Type Conversion/1
  Regen_Direct_Calculation/1(torque) -> [Regen_Available_Torque_Cmd]
  Chart/6(driving) -> [driving]
  inv_state_len/1 -> MATLAB Function3/2(length)
  lat accel/1 -> TC Controller/2(Lateral Accel)
  Ki: 0-1000/1 -> TC Controller/7(Ki)
  MATLAB Function6/1(torque) -> [Driver_Torque]  "Driver Input"
  Switch3/1 -> Multiport Switch/5
  APPS2_OP/1 -> MATLAB Function9/5(APPS2_OP)
  Turn Speeds/2(Out-Speed) -> Out-Speed/1
  [Knob2] -> Min Torque %: 0.0-72.5/1
  MATLAB Function11/2(bpt_r_bar) -> [bpt_r]
  [bpt_f] -> Chart1/2(bpt_f)
  Rate Transition2/1 -> Turn Speeds/1(Lateral Force)
  [TC_Cmd] -> Min/2
  [Brake_Light] -> RT4/1
  Velocity Timestamp/1 -> Kalman Filter/3(Velocity Timestamp)
  [pedals] -> Chart1/4(pedals)
  Regen_switch/1 -> MATLAB Function12/3(Regen_switch), [Regen_Switch]
  [Knob1] -> Power Limiting/1(In1)
  Constant2/1 -> TC Controller/8(Min Torque)
  [bpt_r] -> Chart1/3(bpt_r)
  Min2/1 -> Switch1/3
  inv_en/1 -> MATLAB Function3/1(inv)
  [Fwd_Speed_Est] -> Rate Transition1/1
  DC_Bus_Voltage/1 -> Chart1/5(voltage), [DC_BUS_Voltage]
  MATLAB Function12/2(mcu_input_ctrl) -> mcu_input_ctrl/1, [mcu_input_ctrl]
  Rate Transition1/1 -> Turn Speeds/2(Forward Speed)
  RT3/1 -> Chart/2(RTD_Button)
  [bpt_r] -> Regen_Direct_Calculation/2(BPT_r)
  [Knob1] -> Mu: 0.45-1.7/1
  BMS_IN/1 -> MATLAB Function8/1(bms)
  Screen Button/1 -> Motec Screen/1(Screen Button)
  MATLAB Function7/2(discharge) -> discharge/1
  Turn Speeds/1(In-Speed) -> In-Speed/1
  Accel Report/1 -> Kalman Filter/2(Accel Report)
  wss fl/1 -> Kalman Filter/4(FL)
  Kalman Filter/4(Slip Ratio) -> Slip Ratio/1
  Switch1/1 -> [driver_cmd], driver cmd/1
  Chart/5(inverter_en) -> inverter_en/1
  MATLAB Function7/4(counter) -> counter/1
  ts_state/1 -> MATLAB Function/1(ts)
  Dash Pot 2/1 -> Knob Curve2/1
  apps_sig1/1 -> MATLAB Function9/2(apps_sig1_mcu)
  MATLAB Function7/1(direction) -> direction/1
  TC Controller/3(lights) -> lights/1
  ts_state_len/1 -> MATLAB Function14/2(length), MATLAB Function/2(length)
  MATLAB Function9/2(r_faults) -> [r_faults], r_faults/1
  Chart/4(dc_dc) -> Hit Crossing1/1, Hit Crossing/1
  Chart1/1(Regen_State) -> [Regen_State], Regen_State/1
  inv motor speed/1 -> [INV_Motor_Speed], Subsystem1/3(Motor Speed), Power Limiting/2(In2)
  Driver_Torque_switch/1 -> MATLAB Function12/2(Driver_Torque_switch)
  MATLAB Function8/1(green) -> green light/1
  In26/1 -> Knob Curve3/1
  Dash Pot 1/1 -> Knob Curve1/1
  Kalman Filter/1(Error Covariance) -> Error Covariance/1
  IMD_IN/1 -> MATLAB Function8/2(imd)
  MATLAB Function7/7(torque) -> torque/1
  MATLAB Function7/8(torque_limit) -> torque_limit/1
  bpt_front_1/1 -> MATLAB Function9/1(bpt_sig_mcu), MATLAB Function11/1(bpt_f), MATLAB Function2/1(bpt_f_1)
  MATLAB Function7/6(speed_mode) -> speed_mode/1
  MATLAB Function7/5(speed) -> speed/1
  Lat Accel/1 -> Rate Transition2/1
  Long Accel/1 -> Kalman Filter/1(Accel from CAN)
  MATLAB Function7/3(enable) -> enable/1
  wss rl/1 -> Kalman Filter/6(RL)
  Kalman Filter/3(Forward Speed Estimate) -> Forward Speed Estimate/1, [Fwd_Speed_Est]
  Hit Crossing/1 -> MATLAB Function1/1(on)
  MATLAB Function/1(ts_state) -> RT2/1
  Constant/1 -> dis/1
  radiator/1 -> Subsystem/2(radiator)
  tb_fans/1 -> Subsystem/1(tb_fans)
  Subsystem/2(radiator_fault) -> Mux/1
  Subsystem/1(tb_fans_fault) -> Mux/2
  Mux/1 -> cooling_faults/1
  Hit Crossing1/1 -> MATLAB Function1/2(off)
  MATLAB Function1/1(cooling_out_1) -> cooling_loop/1
  MATLAB Function1/2(cooling_out_2) -> cooling_tb_fans/1
  MATLAB Function1/3(cooling_out_3) -> cooling_radiator/1
  MATLAB Function2/1(bpt_f_1_bar) -> bpt_f_1_bar/1
  MATLAB Function2/2(bpt_f_2_bar) -> bpt_f_2_bar/1
  [Knob3] -> Regen_Direct_Calculation/3(Brake Bias Knob)
  Subsystem1/1(SOC Power Limit) -> Min3/2
  If/1 -> TC Controller/Action
  Rate Transition/1 -> If/1
  [Knob1] -> 1-D Lookup Table3/1
  SDC Sig/1 -> Chart/5(SDC_Sig)
  MATLAB Function/2(time_out) -> out/1, Chart/4(ts_state_timeout)
  [Knob3] -> MATLAB Function5/1(brake_bias)
  MATLAB Function5/1(servo_pos) -> TX/1
  [mcu_input_ctrl] -> MATLAB Function5/2(mcu_control)
  Servo_Pos/1 -> MATLAB Function13/1(pos_raw)
  MATLAB Function13/1(pos) -> brake_bias_pos/1, Equal/1
  Regen Servo Pos/1 -> Equal/2
  Kp: 0-115/1 -> TC Controller/6(Kp)
  Mu: 0.45-1.7/1 -> ?
  GreaterThanOrEqual2/1 -> Out18/1, [Brake_Light]
  Chart/3(buzzer) -> buzzer/1
  Chart/2(ready_led) -> ready_led/1
  Constant4/1 -> Equal1/2
  RTD_Button/1 -> Equal1/1
  BSM Discharge/1 -> MATLAB Function14/1(bsm_discharge)
  [driver_input_ctrl] -> Switch/2
  Switch/1 -> MATLAB Function6/3(TORQUE_MAX)
  Constant5/1 -> Switch/3
  [DC_BUS_Voltage] -> Power Limiting1/1(DC Bus Voltage)
  [INV_Motor_Speed] -> Power Limiting1/2(In2)
  Power Limiting1/1(driver cmd) -> Abs/1
  Abs1/1 -> Min1/1
  Abs/1 -> Min1/2
  Min1/1 -> Product/2
  Sign/1 -> Product/1
  Product/1 -> MATLAB Function7/2(pedal_torque)
  INV Id/1 -> Power Limiting1/3(INV Id)
  INV Iq/1 -> Power Limiting1/4(INV Iq)
  MATLAB Function8/2(red) -> AND/2
  AND/1 -> red light/1
  DC Bus Current/1 -> [DC_Bus_Current], Power Limiting1/5(DC Bus Current)
  Constant6/1 -> Chart1/7(brake_bias_good)
  [DC_Bus_Current] -> Chart/8(DC_Bus_Current)
  [Model_Cmd] -> TC Torque Cmd/1
  BMS Min Voltage/1 -> Power Limiting1/7(BMS Min Voltage)
  Constant7/1 -> MATLAB Function12/1(TC_switch)
  [TC_switch] -> Power Limiting1/8(Switch)
  [Knob2] -> Power Limiting1/9(Current Lim Knob)
